simulink model "leantest"  (R2016b)
settings: Solver=FixedStepAuto  StartTime=0.0  StopTime=1  FixedStep=0.001  RelTol=1e-3
settings Model: Creator=labuser  LastModifiedBy=labuser

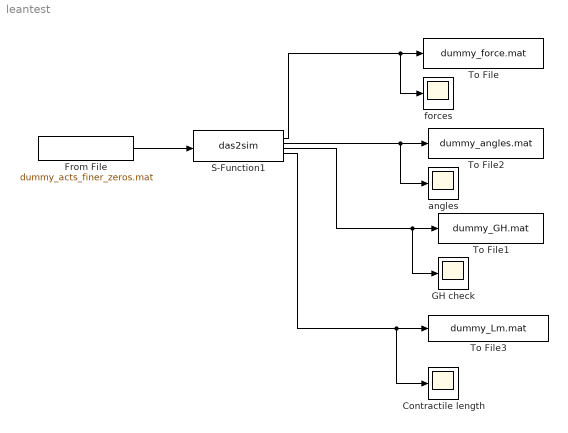
== system leantest ==
  Contractile length : Scope
  From File : FromFile  FileName=dummy_acts_finer_zeros.mat  OutDataTypeStr=double  SampleTime=0.001
  GH check : Scope
  S-Function1 : S-Function  FunctionName=das2sim  Parameters=[0;0;0]  SFunctionDeploymentMode=off  EnableBusSupport=off
  To File : ToFile  Filename=dummy_force.mat
  To File1 : ToFile  Filename=dummy_GH.mat
  To File2 : ToFile  Filename=dummy_angles.mat
  To File3 : ToFile  Filename=dummy_Lm.mat
  angles : Scope
  forces : Scope
  wires:
  S-Function1/4 -> Contractile length/1, To File3/1
  From File/1 -> S-Function1/1
  S-Function1/1 -> forces/1, To File/1
  S-Function1/2 -> angles/1, To File2/1
  S-Function1/3 -> GH check/1, To File1/1
